simulink model "Q2"  (R2022b)
settings: Solver=VariableStepAuto  StartTime=0.0  StopTime=10.0  RelTol=1e-3
settings Model: Creator=Ali  LastModifiedBy=Ali

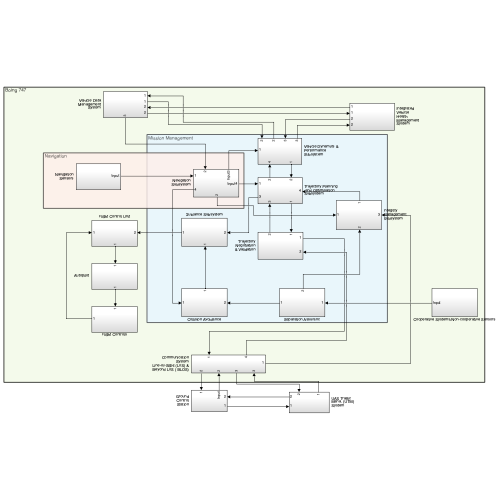
[thumbnail: Simulink's stored preview of the top-level diagram]
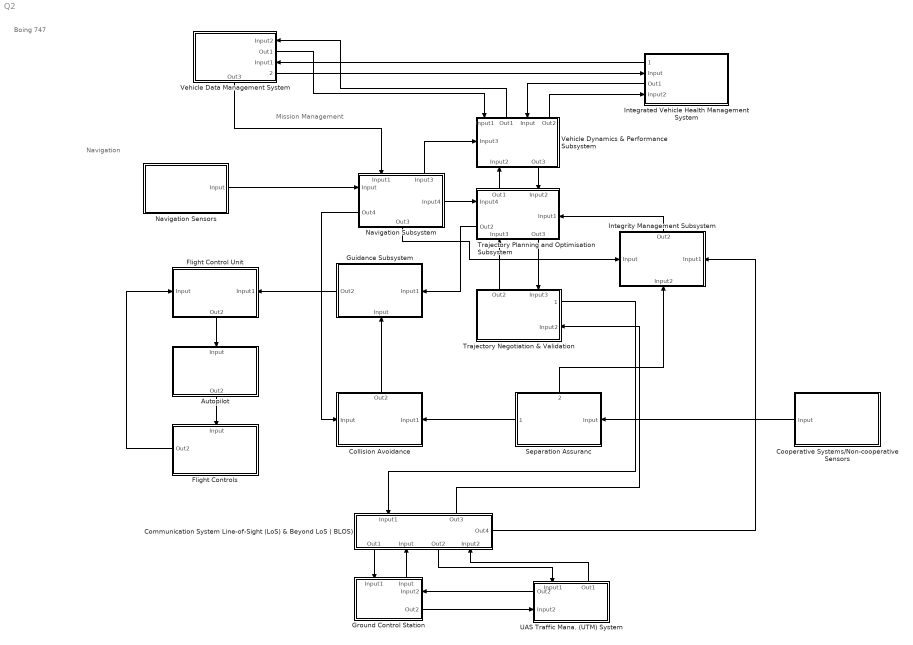
== system Q2 ==
  note: Mission Management
  note: Navigation
  note: Boing 747
  Autopilot : Subsystem
      settings: PortSchema="{\"entries\":[{\"content\":{\"sides\":[{\"content\":{\"connectorIds\":[]},\"type\":\"ConnectorPlacement.EquallySpacedRectSide\",\"uuid\":\"7c03228e-e6de-4210-83e4-dc60ea5d03ec\"},{\"content\":{\"connectorIds\":[],\"side\":\"RIGHT\"},\"type\":\"ConnectorPlacement.EquallySpacedRectSide\",\"uuid\":\"398f5b5b-7985-47d4-80b4-f710280625a6\"},{\"content\":{\"connectorIds\":[\"In1\"],\"side\":\"TOP\"},\"type\":\"ConnectorPlacement.EquallySpacedRectSide\",\"uuid\":\"212a440f-1f73-46c7-990f-e1425be29cd1\"},{\"content\":{\"connectorIds\":[\"Out1\"],\"side\":\"BOTTOM\"},\"type\":\"ConnectorPlacement.EquallySpacedRectSide\",\"uuid\":\"b57b75e4-92e7-45b5-b420-ccd9edaba603\"}]},\"type\":\"ConnectorPlacement.EquallySpacedConnector\",\"uuid\":\"cb83deef-b6b8-410a-b432-b2f3f2a9e8ae\"}],\"packageUris\":[\"http://schema.mathworks.com/mf0/Connector/R2020b\"],\"version\":\"1.0\"}"
  Collision Avoidance : Subsystem
      settings: PortSchema="{\"entries\":[{\"content\":{\"sides\":[{\"content\":{\"connectorIds\":[\"In1\"]},\"type\":\"ConnectorPlacement.EquallySpacedRectSide\",\"uuid\":\"8816de1e-4171-47af-bbd0-c7093bdd2ec4\"},{\"content\":{\"connectorIds\":[\"In2\"],\"side\":\"RIGHT\"},\"type\":\"ConnectorPlacement.EquallySpacedRectSide\",\"uuid\":\"4ec5b307-27a2-4754-b3e3-e34b35b208c2\"},{\"content\":{\"connectorIds\":[\"Out1\"],\"side\":\"TOP\"},\"type\":\"ConnectorPlacement.EquallySpacedRectSide\",\"uuid\":\"1be75602-f59e-4616-8d3b-3f7c07037b2b\"},{\"content\":{\"connectorIds\":[],\"side\":\"BOTTOM\"},\"type\":\"ConnectorPlacement.EquallySpacedRectSide\",\"uuid\":\"aaca4339-a36b-4f6c-91d5-5c0f7e0a86f3\"}]},\"type\":\"ConnectorPlacement.EquallySpacedConnector\",\"uuid\":\"f2ce33cf-07fa-49b4-80b6-e618028f6f8d\"}],\"packageUris\":[\"http://schema.mathworks.com/mf0/Connector/R2020b\"],\"version\":\"1.0\"}"
  Communication System Line-of-Sight (LoS) & Beyond LoS ( BLOS) : Subsystem
      settings: PortSchema="{\"entries\":[{\"content\":{\"sides\":[{\"content\":{\"connectorIds\":[]},\"type\":\"ConnectorPlacement.EquallySpacedRectSide\",\"uuid\":\"8816de1e-4171-47af-bbd0-c7093bdd2ec4\"},{\"content\":{\"connectorIds\":[\"Out1\"],\"side\":\"RIGHT\"},\"type\":\"ConnectorPlacement.EquallySpacedRectSide\",\"uuid\":\"4ec5b307-27a2-4754-b3e3-e34b35b208c2\"},{\"content\":{\"connectorIds\":[\"In1\",\"Out4\"],\"side\":\"TOP\"},\"type\":\"ConnectorPlacement.EquallySpacedRectSide\",\"uuid\":\"1be75602-f59e-4616-8d3b-3f7c07037b2b\"},{\"content\":{\"connectorIds\":[\"Out2\",\"In2\",\"Out3\",\"In3\"],\"side\":\"BOTTOM\"},\"type\":\"ConnectorPlacement.EquallySpacedRectSide\",\"uuid\":\"aaca4339-a36b-4f6c-91d5-5c0f7e0a86f3\"}]},\"type\":\"ConnectorPlacement.EquallySpacedConnector\",\"uuid\":\"f2ce33cf-07fa-49b4-80b6-e618028f6f8d\"}],\"packageUris\":[\"http://schema.mathworks.com/mf0/Connector/R2020b\"],\"version\":\"1.0\"}"
  Cooperative Systems/Non-cooperative Sensors : Subsystem
      settings: PortSchema="{\"entries\":[{\"content\":{\"sides\":[{\"content\":{\"connectorIds\":[\"Out1\"]},\"type\":\"ConnectorPlacement.EquallySpacedRectSide\",\"uuid\":\"8816de1e-4171-47af-bbd0-c7093bdd2ec4\"},{\"content\":{\"connectorIds\":[],\"side\":\"RIGHT\"},\"type\":\"ConnectorPlacement.EquallySpacedRectSide\",\"uuid\":\"4ec5b307-27a2-4754-b3e3-e34b35b208c2\"},{\"content\":{\"connectorIds\":[],\"side\":\"TOP\"},\"type\":\"ConnectorPlacement.EquallySpacedRectSide\",\"uuid\":\"1be75602-f59e-4616-8d3b-3f7c07037b2b\"},{\"content\":{\"connectorIds\":[],\"side\":\"BOTTOM\"},\"type\":\"ConnectorPlacement.EquallySpacedRectSide\",\"uuid\":\"aaca4339-a36b-4f6c-91d5-5c0f7e0a86f3\"}]},\"type\":\"ConnectorPlacement.EquallySpacedConnector\",\"uuid\":\"f2ce33cf-07fa-49b4-80b6-e618028f6f8d\"}],\"packageUris\":[\"http://schema.mathworks.com/mf0/Connector/R2020b\"],\"version\":\"1.0\"}"
  Flight Control Unit : Subsystem
      settings: PortSchema="{\"entries\":[{\"content\":{\"sides\":[{\"content\":{\"connectorIds\":[\"In1\"]},\"type\":\"ConnectorPlacement.EquallySpacedRectSide\",\"uuid\":\"7c03228e-e6de-4210-83e4-dc60ea5d03ec\"},{\"content\":{\"connectorIds\":[\"In2\"],\"side\":\"RIGHT\"},\"type\":\"ConnectorPlacement.EquallySpacedRectSide\",\"uuid\":\"398f5b5b-7985-47d4-80b4-f710280625a6\"},{\"content\":{\"connectorIds\":[],\"side\":\"TOP\"},\"type\":\"ConnectorPlacement.EquallySpacedRectSide\",\"uuid\":\"212a440f-1f73-46c7-990f-e1425be29cd1\"},{\"content\":{\"connectorIds\":[\"Out1\"],\"side\":\"BOTTOM\"},\"type\":\"ConnectorPlacement.EquallySpacedRectSide\",\"uuid\":\"b57b75e4-92e7-45b5-b420-ccd9edaba603\"}]},\"type\":\"ConnectorPlacement.EquallySpacedConnector\",\"uuid\":\"cb83deef-b6b8-410a-b432-b2f3f2a9e8ae\"}],\"packageUris\":[\"http://schema.mathworks.com/mf0/Connector/R2020b\"],\"version\":\"1.0\"}"
  Flight Controls : Subsystem
      settings: PortSchema="{\"entries\":[{\"content\":{\"sides\":[{\"content\":{\"connectorIds\":[\"Out1\"]},\"type\":\"ConnectorPlacement.EquallySpacedRectSide\",\"uuid\":\"7c03228e-e6de-4210-83e4-dc60ea5d03ec\"},{\"content\":{\"connectorIds\":[],\"side\":\"RIGHT\"},\"type\":\"ConnectorPlacement.EquallySpacedRectSide\",\"uuid\":\"398f5b5b-7985-47d4-80b4-f710280625a6\"},{\"content\":{\"connectorIds\":[\"In1\"],\"side\":\"TOP\"},\"type\":\"ConnectorPlacement.EquallySpacedRectSide\",\"uuid\":\"212a440f-1f73-46c7-990f-e1425be29cd1\"},{\"content\":{\"connectorIds\":[],\"side\":\"BOTTOM\"},\"type\":\"ConnectorPlacement.EquallySpacedRectSide\",\"uuid\":\"b57b75e4-92e7-45b5-b420-ccd9edaba603\"}]},\"type\":\"ConnectorPlacement.EquallySpacedConnector\",\"uuid\":\"cb83deef-b6b8-410a-b432-b2f3f2a9e8ae\"}],\"packageUris\":[\"http://schema.mathworks.com/mf0/Connector/R2020b\"],\"version\":\"1.0\"}"
  Ground Control Station : Subsystem
      settings: PortSchema="{\"entries\":[{\"content\":{\"sides\":[{\"content\":{\"connectorIds\":[]},\"type\":\"ConnectorPlacement.EquallySpacedRectSide\",\"uuid\":\"8816de1e-4171-47af-bbd0-c7093bdd2ec4\"},{\"content\":{\"connectorIds\":[\"In2\",\"Out1\"],\"side\":\"RIGHT\"},\"type\":\"ConnectorPlacement.EquallySpacedRectSide\",\"uuid\":\"4ec5b307-27a2-4754-b3e3-e34b35b208c2\"},{\"content\":{\"connectorIds\":[\"In1\",\"Out2\"],\"side\":\"TOP\"},\"type\":\"ConnectorPlacement.EquallySpacedRectSide\",\"uuid\":\"1be75602-f59e-4616-8d3b-3f7c07037b2b\"},{\"content\":{\"connectorIds\":[],\"side\":\"BOTTOM\"},\"type\":\"ConnectorPlacement.EquallySpacedRectSide\",\"uuid\":\"aaca4339-a36b-4f6c-91d5-5c0f7e0a86f3\"}]},\"type\":\"ConnectorPlacement.EquallySpacedConnector\",\"uuid\":\"f2ce33cf-07fa-49b4-80b6-e618028f6f8d\"}],\"packageUris\":[\"http://schema.mathworks.com/mf0/Connector/R2020b\"],\"version\":\"1.0\"}"
  Guidance Subsystem : Subsystem
      settings: PortSchema="{\"entries\":[{\"content\":{\"sides\":[{\"content\":{\"connectorIds\":[\"Out1\"]},\"type\":\"ConnectorPlacement.EquallySpacedRectSide\",\"uuid\":\"8816de1e-4171-47af-bbd0-c7093bdd2ec4\"},{\"content\":{\"connectorIds\":[\"In2\"],\"side\":\"RIGHT\"},\"type\":\"ConnectorPlacement.EquallySpacedRectSide\",\"uuid\":\"4ec5b307-27a2-4754-b3e3-e34b35b208c2\"},{\"content\":{\"connectorIds\":[],\"side\":\"TOP\"},\"type\":\"ConnectorPlacement.EquallySpacedRectSide\",\"uuid\":\"1be75602-f59e-4616-8d3b-3f7c07037b2b\"},{\"content\":{\"connectorIds\":[\"In1\"],\"side\":\"BOTTOM\"},\"type\":\"ConnectorPlacement.EquallySpacedRectSide\",\"uuid\":\"aaca4339-a36b-4f6c-91d5-5c0f7e0a86f3\"}]},\"type\":\"ConnectorPlacement.EquallySpacedConnector\",\"uuid\":\"f2ce33cf-07fa-49b4-80b6-e618028f6f8d\"}],\"packageUris\":[\"http://schema.mathworks.com/mf0/Connector/R2020b\"],\"version\":\"1.0\"}"
  Integrated Vehicle Health Management System : Subsystem
      settings: PortSchema="{\"entries\":[{\"content\":{\"sides\":[{\"content\":{\"connectorIds\":[\"Out1\",\"In1\",\"Out2\",\"In2\"]},\"type\":\"ConnectorPlacement.EquallySpacedRectSide\",\"uuid\":\"bd36125d-75c5-4143-b99c-3e4a87d10701\"},{\"content\":{\"connectorIds\":[],\"side\":\"RIGHT\"},\"type\":\"ConnectorPlacement.EquallySpacedRectSide\",\"uuid\":\"e6754b16-36a5-4be2-b98d-b46917597dce\"},{\"content\":{\"connectorIds\":[],\"side\":\"TOP\"},\"type\":\"ConnectorPlacement.EquallySpacedRectSide\",\"uuid\":\"193bbe33-aa7f-43da-961a-60435cc2b4dc\"},{\"content\":{\"connectorIds\":[],\"side\":\"BOTTOM\"},\"type\":\"ConnectorPlacement.EquallySpacedRectSide\",\"uuid\":\"1a0f7017-b5e6-4739-a088-f50189ea50e9\"}]},\"type\":\"ConnectorPlacement.EquallySpacedConnector\",\"uuid\":\"e77c47bd-b0a0-4c61-ab2d-e4f8b97a4182\"}],\"packageUris\":[\"http://schema.mathworks.com/mf0/Connector/R2020b\"],\"version\":\"1.0\"}"
  Integrity Management Subsystem : Subsystem
      settings: PortSchema="{\"entries\":[{\"content\":{\"sides\":[{\"content\":{\"connectorIds\":[\"In1\"]},\"type\":\"ConnectorPlacement.EquallySpacedRectSide\",\"uuid\":\"8816de1e-4171-47af-bbd0-c7093bdd2ec4\"},{\"content\":{\"connectorIds\":[\"In3\"],\"side\":\"RIGHT\"},\"type\":\"ConnectorPlacement.EquallySpacedRectSide\",\"uuid\":\"4ec5b307-27a2-4754-b3e3-e34b35b208c2\"},{\"content\":{\"connectorIds\":[\"Out1\"],\"side\":\"TOP\"},\"type\":\"ConnectorPlacement.EquallySpacedRectSide\",\"uuid\":\"1be75602-f59e-4616-8d3b-3f7c07037b2b\"},{\"content\":{\"connectorIds\":[\"In2\"],\"side\":\"BOTTOM\"},\"type\":\"ConnectorPlacement.EquallySpacedRectSide\",\"uuid\":\"aaca4339-a36b-4f6c-91d5-5c0f7e0a86f3\"}]},\"type\":\"ConnectorPlacement.EquallySpacedConnector\",\"uuid\":\"f2ce33cf-07fa-49b4-80b6-e618028f6f8d\"}],\"packageUris\":[\"http://schema.mathworks.com/mf0/Connector/R2020b\"],\"version\":\"1.0\"}"
  Navigation Subsystem : Subsystem
      settings: PortSchema="{\"entries\":[{\"content\":{\"sides\":[{\"content\":{\"connectorIds\":[\"In1\",\"Out4\"]},\"type\":\"ConnectorPlacement.EquallySpacedRectSide\",\"uuid\":\"8816de1e-4171-47af-bbd0-c7093bdd2ec4\"},{\"content\":{\"connectorIds\":[\"Out1\"],\"side\":\"RIGHT\"},\"type\":\"ConnectorPlacement.EquallySpacedRectSide\",\"uuid\":\"4ec5b307-27a2-4754-b3e3-e34b35b208c2\"},{\"content\":{\"connectorIds\":[\"In2\",\"Out3\"],\"side\":\"TOP\"},\"type\":\"ConnectorPlacement.EquallySpacedRectSide\",\"uuid\":\"1be75602-f59e-4616-8d3b-3f7c07037b2b\"},{\"content\":{\"connectorIds\":[\"Out2\"],\"side\":\"BOTTOM\"},\"type\":\"ConnectorPlacement.EquallySpacedRectSide\",\"uuid\":\"aaca4339-a36b-4f6c-91d5-5c0f7e0a86f3\"}]},\"type\":\"ConnectorPlacement.EquallySpacedConnector\",\"uuid\":\"f2ce33cf-07fa-49b4-80b6-e618028f6f8d\"}],\"packageUris\":[\"http://schema.mathworks.com/mf0/Connector/R2020b\"],\"version\":\"1.0\"}"
  Navigation Sensors : Subsystem
  Separation Assuranc : Subsystem
      settings: PortSchema="{\"entries\":[{\"content\":{\"sides\":[{\"content\":{\"connectorIds\":[\"Out2\"]},\"type\":\"ConnectorPlacement.EquallySpacedRectSide\",\"uuid\":\"8816de1e-4171-47af-bbd0-c7093bdd2ec4\"},{\"content\":{\"connectorIds\":[\"In1\"],\"side\":\"RIGHT\"},\"type\":\"ConnectorPlacement.EquallySpacedRectSide\",\"uuid\":\"4ec5b307-27a2-4754-b3e3-e34b35b208c2\"},{\"content\":{\"connectorIds\":[\"Out1\"],\"side\":\"TOP\"},\"type\":\"ConnectorPlacement.EquallySpacedRectSide\",\"uuid\":\"1be75602-f59e-4616-8d3b-3f7c07037b2b\"},{\"content\":{\"connectorIds\":[],\"side\":\"BOTTOM\"},\"type\":\"ConnectorPlacement.EquallySpacedRectSide\",\"uuid\":\"aaca4339-a36b-4f6c-91d5-5c0f7e0a86f3\"}]},\"type\":\"ConnectorPlacement.EquallySpacedConnector\",\"uuid\":\"f2ce33cf-07fa-49b4-80b6-e618028f6f8d\"}],\"packageUris\":[\"http://schema.mathworks.com/mf0/Connector/R2020b\"],\"version\":\"1.0\"}"
  Trajectory Negotiation & Validation : Subsystem
      settings: PortSchema="{\"entries\":[{\"content\":{\"sides\":[{\"content\":{\"connectorIds\":[]},\"type\":\"ConnectorPlacement.EquallySpacedRectSide\",\"uuid\":\"bd36125d-75c5-4143-b99c-3e4a87d10701\"},{\"content\":{\"connectorIds\":[\"Out1\",\"In2\"],\"side\":\"RIGHT\"},\"type\":\"ConnectorPlacement.EquallySpacedRectSide\",\"uuid\":\"e6754b16-36a5-4be2-b98d-b46917597dce\"},{\"content\":{\"connectorIds\":[\"Out2\",\"In1\"],\"side\":\"TOP\"},\"type\":\"ConnectorPlacement.EquallySpacedRectSide\",\"uuid\":\"193bbe33-aa7f-43da-961a-60435cc2b4dc\"},{\"content\":{\"connectorIds\":[],\"side\":\"BOTTOM\"},\"type\":\"ConnectorPlacement.EquallySpacedRectSide\",\"uuid\":\"1a0f7017-b5e6-4739-a088-f50189ea50e9\"}]},\"type\":\"ConnectorPlacement.EquallySpacedConnector\",\"uuid\":\"e77c47bd-b0a0-4c61-ab2d-e4f8b97a4182\"}],\"packageUris\":[\"http://schema.mathworks.com/mf0/Connector/R2020b\"],\"version\":\"1.0\"}"
  Trajectory Planning and Optimisation Subsystem : Subsystem
      settings: PortSchema="{\"entries\":[{\"content\":{\"sides\":[{\"content\":{\"connectorIds\":[\"In1\",\"Out3\"]},\"type\":\"ConnectorPlacement.EquallySpacedRectSide\",\"uuid\":\"bd36125d-75c5-4143-b99c-3e4a87d10701\"},{\"content\":{\"connectorIds\":[\"In4\"],\"side\":\"RIGHT\"},\"type\":\"ConnectorPlacement.EquallySpacedRectSide\",\"uuid\":\"e6754b16-36a5-4be2-b98d-b46917597dce\"},{\"content\":{\"connectorIds\":[\"Out2\",\"In2\"],\"side\":\"TOP\"},\"type\":\"ConnectorPlacement.EquallySpacedRectSide\",\"uuid\":\"193bbe33-aa7f-43da-961a-60435cc2b4dc\"},{\"content\":{\"connectorIds\":[\"In3\",\"Out1\"],\"side\":\"BOTTOM\"},\"type\":\"ConnectorPlacement.EquallySpacedRectSide\",\"uuid\":\"1a0f7017-b5e6-4739-a088-f50189ea50e9\"}]},\"type\":\"ConnectorPlacement.EquallySpacedConnector\",\"uuid\":\"e77c47bd-b0a0-4c61-ab2d-e4f8b97a4182\"}],\"packageUris\":[\"http://schema.mathworks.com/mf0/Connector/R2020b\"],\"version\":\"1.0\"}"
  UAS Traffic Mana. (UTM) System : Subsystem
      settings: PortSchema="{\"entries\":[{\"content\":{\"sides\":[{\"content\":{\"connectorIds\":[\"Out2\",\"In1\"]},\"type\":\"ConnectorPlacement.EquallySpacedRectSide\",\"uuid\":\"8816de1e-4171-47af-bbd0-c7093bdd2ec4\"},{\"content\":{\"connectorIds\":[],\"side\":\"RIGHT\"},\"type\":\"ConnectorPlacement.EquallySpacedRectSide\",\"uuid\":\"4ec5b307-27a2-4754-b3e3-e34b35b208c2\"},{\"content\":{\"connectorIds\":[\"In2\",\"Out1\"],\"side\":\"TOP\"},\"type\":\"ConnectorPlacement.EquallySpacedRectSide\",\"uuid\":\"1be75602-f59e-4616-8d3b-3f7c07037b2b\"},{\"content\":{\"connectorIds\":[],\"side\":\"BOTTOM\"},\"type\":\"ConnectorPlacement.EquallySpacedRectSide\",\"uuid\":\"aaca4339-a36b-4f6c-91d5-5c0f7e0a86f3\"}]},\"type\":\"ConnectorPlacement.EquallySpacedConnector\",\"uuid\":\"f2ce33cf-07fa-49b4-80b6-e618028f6f8d\"}],\"packageUris\":[\"http://schema.mathworks.com/mf0/Connector/R2020b\"],\"version\":\"1.0\"}"
  Vehicle Data Management System : Subsystem
      settings: PortSchema="{\"entries\":[{\"content\":{\"sides\":[{\"content\":{\"connectorIds\":[]},\"type\":\"ConnectorPlacement.EquallySpacedRectSide\",\"uuid\":\"bd36125d-75c5-4143-b99c-3e4a87d10701\"},{\"content\":{\"connectorIds\":[\"In1\",\"Out1\",\"In2\",\"Out2\"],\"side\":\"RIGHT\"},\"type\":\"ConnectorPlacement.EquallySpacedRectSide\",\"uuid\":\"e6754b16-36a5-4be2-b98d-b46917597dce\"},{\"content\":{\"connectorIds\":[],\"side\":\"TOP\"},\"type\":\"ConnectorPlacement.EquallySpacedRectSide\",\"uuid\":\"193bbe33-aa7f-43da-961a-60435cc2b4dc\"},{\"content\":{\"connectorIds\":[\"Out3\"],\"side\":\"BOTTOM\"},\"type\":\"ConnectorPlacement.EquallySpacedRectSide\",\"uuid\":\"1a0f7017-b5e6-4739-a088-f50189ea50e9\"}]},\"type\":\"ConnectorPlacement.EquallySpacedConnector\",\"uuid\":\"e77c47bd-b0a0-4c61-ab2d-e4f8b97a4182\"}],\"packageUris\":[\"http://schema.mathworks.com/mf0/Connector/R2020b\"],\"version\":\"1.0\"}"
  Vehicle Dynamics & Performance Subsystem : Subsystem
      settings: PortSchema="{\"entries\":[{\"content\":{\"sides\":[{\"content\":{\"connectorIds\":[\"In1\"]},\"type\":\"ConnectorPlacement.EquallySpacedRectSide\",\"uuid\":\"bd36125d-75c5-4143-b99c-3e4a87d10701\"},{\"content\":{\"connectorIds\":[],\"side\":\"RIGHT\"},\"type\":\"ConnectorPlacement.EquallySpacedRectSide\",\"uuid\":\"e6754b16-36a5-4be2-b98d-b46917597dce\"},{\"content\":{\"connectorIds\":[\"In2\",\"Out2\",\"In3\",\"Out3\"],\"side\":\"TOP\"},\"type\":\"ConnectorPlacement.EquallySpacedRectSide\",\"uuid\":\"193bbe33-aa7f-43da-961a-60435cc2b4dc\"},{\"content\":{\"connectorIds\":[\"In4\",\"Out1\"],\"side\":\"BOTTOM\"},\"type\":\"ConnectorPlacement.EquallySpacedRectSide\",\"uuid\":\"1a0f7017-b5e6-4739-a088-f50189ea50e9\"}]},\"type\":\"ConnectorPlacement.EquallySpacedConnector\",\"uuid\":\"e77c47bd-b0a0-4c61-ab2d-e4f8b97a4182\"}],\"packageUris\":[\"http://schema.mathworks.com/mf0/Connector/R2020b\"],\"version\":\"1.0\"}"
  wires:
  Vehicle Dynamics & Performance Subsystem/3(Out2) -> Integrated Vehicle Health Management System/2(Input2)
  Integrated Vehicle Health Management System/2(Out1) -> Vehicle Dynamics & Performance Subsystem/3(Input)
  Vehicle Dynamics & Performance Subsystem/2(Out1) -> Vehicle Data Management System/1(Input2)
  Vehicle Data Management System/1(Out1) -> Vehicle Dynamics & Performance Subsystem/2(Input1)
  Vehicle Dynamics & Performance Subsystem/1(Out3) -> Trajectory Planning and Optimisation Subsystem/2(Input2)
  Trajectory Planning and Optimisation Subsystem/2(Out1) -> Vehicle Dynamics & Performance Subsystem/4(Input2)
  Navigation Subsystem/1(Input4) -> Trajectory Planning and Optimisation Subsystem/1(Input4)
  Navigation Subsystem/3(Input3) -> Vehicle Dynamics & Performance Subsystem/1(Input3)
  Vehicle Data Management System/3(Out3) -> Navigation Subsystem/2(Input1)
  Trajectory Planning and Optimisation Subsystem/3(Out2) -> Guidance Subsystem/2(Input1)
  Navigation Subsystem/2(Out3) -> Integrity Management Subsystem/1(Input)
  Navigation Sensors/1(Input) -> Navigation Subsystem/1(Input)
  Navigation Subsystem/4(Out4) -> Collision Avoidance/1(Input)
  Guidance Subsystem/1(Out2) -> Flight Control Unit/2(Input1)
  Flight Controls/1(Out2) -> Flight Control Unit/1(Input)
  Flight Control Unit/1(Out2) -> Autopilot/1(Input)
  Autopilot/1(Out2) -> Flight Controls/1(Input)
  Collision Avoidance/1(Out2) -> Guidance Subsystem/1(Input)
  Separation Assuranc/2(1) -> Collision Avoidance/2(Input1)
  Separation Assuranc/1(2) -> Integrity Management Subsystem/2(Input2)
  Cooperative Systems/Non-cooperative Sensors/1(Input) -> Separation Assuranc/1(Input)
  Ground Control Station/2(Input) -> Communication System Line-of-Sight (LoS) & Beyond LoS ( BLOS)/2(Input)
  Communication System Line-of-Sight (LoS) & Beyond LoS ( BLOS)/2(Out1) -> Ground Control Station/1(Input1)
  Communication System Line-of-Sight (LoS) & Beyond LoS ( BLOS)/3(Out2) -> UAS Traffic Mana. (UTM) System/2(Input1)
  UAS Traffic Mana. (UTM) System/1(Out1) -> Communication System Line-of-Sight (LoS) & Beyond LoS ( BLOS)/3(Input2)
  UAS Traffic Mana. (UTM) System/2(Out2) -> Ground Control Station/2(Input2)
  Ground Control Station/1(Out2) -> UAS Traffic Mana. (UTM) System/1(Input2)
  Communication System Line-of-Sight (LoS) & Beyond LoS ( BLOS)/4(Out3) -> Trajectory Negotiation & Validation/2(Input2)
  Trajectory Negotiation & Validation/1(1) -> Communication System Line-of-Sight (LoS) & Beyond LoS ( BLOS)/1(Input1)
  Trajectory Planning and Optimisation Subsystem/1(Out3) -> Trajectory Negotiation & Validation/1(Input3)
  Trajectory Negotiation & Validation/2(Out2) -> Trajectory Planning and Optimisation Subsystem/3(Input3)
  Vehicle Data Management System/2(2) -> Integrated Vehicle Health Management System/1(Input)
  Communication System Line-of-Sight (LoS) & Beyond LoS ( BLOS)/1(Out4) -> Integrity Management Subsystem/3(Input1)
  Integrity Management Subsystem/1(Out2) -> Trajectory Planning and Optimisation Subsystem/4(Input1)
  Integrated Vehicle Health Management System/1(1) -> Vehicle Data Management System/2(Input1)

== system Q2/Autopilot ==
  Input : Inport
  Out2 : Outport
  wires:
  Input/1 -> Out2/1

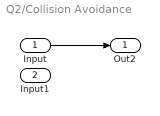
== system Q2/Collision Avoidance ==
  Input : Inport
  Input1 : Inport  Port=2
  Out2 : Outport
  wires:
  Input/1 -> Out2/1

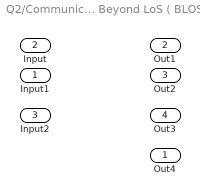
== system Q2/Communication System Line-of-Sight (LoS) & Beyond LoS ( BLOS) ==
  Input1 : Inport
  Input : Inport  Port=2
  Input2 : Inport  Port=3
  Out4 : Outport
  Out1 : Outport  Port=2
  Out2 : Outport  Port=3
  Out3 : Outport  Port=4

== system Q2/Cooperative Systems//Non-cooperative Sensors ==
  Input : Outport

== system Q2/Flight Control Unit ==
  Input : Inport
  Input1 : Inport  Port=2
  Out2 : Outport
  wires:
  Input/1 -> Out2/1

== system Q2/Flight Controls ==
  Input : Inport
  Out2 : Outport
  wires:
  Input/1 -> Out2/1

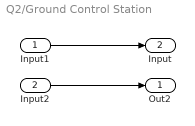
== system Q2/Ground Control Station ==
  Input1 : Inport
  Input2 : Inport  Port=2
  Out2 : Outport
  Input : Outport  Port=2
  wires:
  Input1/1 -> Input/1
  Input2/1 -> Out2/1

== system Q2/Guidance Subsystem ==
  Input : Inport
  Input1 : Inport  Port=2
  Out2 : Outport
  wires:
  Input/1 -> Out2/1

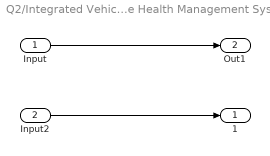
== system Q2/Integrated Vehicle Health Management System ==
  Input : Inport
  Input2 : Inport  Port=2
  1 : Outport
  Out1 : Outport  Port=2
  wires:
  Input/1 -> Out1/1
  Input2/1 -> 1/1

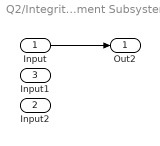
== system Q2/Integrity Management Subsystem ==
  Input : Inport
  Input2 : Inport  Port=2
  Input1 : Inport  Port=3
  Out2 : Outport
  wires:
  Input/1 -> Out2/1

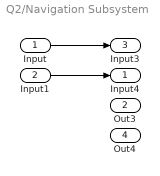
== system Q2/Navigation Subsystem ==
  Input : Inport
  Input1 : Inport  Port=2
  Input4 : Outport
  Out3 : Outport  Port=2
  Input3 : Outport  Port=3
  Out4 : Outport  Port=4
  wires:
  Input1/1 -> Input4/1
  Input/1 -> Input3/1

== system Q2/Navigation Sensors ==
  Input : Outport

== system Q2/Separation Assuranc ==
  Input : Inport
  2 : Outport
  1 : Outport  Port=2
  wires:
  Input/1 -> 1/1

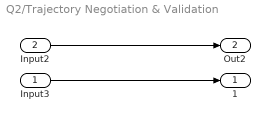
== system Q2/Trajectory Negotiation & Validation ==
  Input3 : Inport
  Input2 : Inport  Port=2
  1 : Outport
  Out2 : Outport  Port=2
  wires:
  Input2/1 -> Out2/1
  Input3/1 -> 1/1

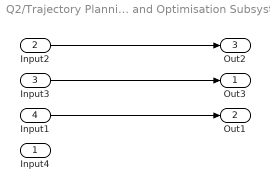
== system Q2/Trajectory Planning and Optimisation Subsystem ==
  Input4 : Inport
  Input2 : Inport  Port=2
  Input3 : Inport  Port=3
  Input1 : Inport  Port=4
  Out3 : Outport
  Out1 : Outport  Port=2
  Out2 : Outport  Port=3
  wires:
  Input2/1 -> Out2/1
  Input3/1 -> Out3/1
  Input1/1 -> Out1/1

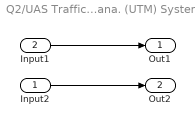
== system Q2/UAS Traffic Mana. (UTM) System ==
  Input2 : Inport
  Input1 : Inport  Port=2
  Out1 : Outport
  Out2 : Outport  Port=2
  wires:
  Input1/1 -> Out1/1
  Input2/1 -> Out2/1

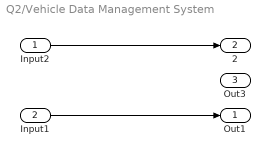
== system Q2/Vehicle Data Management System ==
  Input2 : Inport
  Input1 : Inport  Port=2
  Out1 : Outport
  2 : Outport  Port=2
  Out3 : Outport  Port=3
  wires:
  Input2/1 -> 2/1
  Input1/1 -> Out1/1

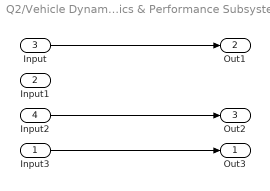
== system Q2/Vehicle Dynamics & Performance Subsystem ==
  Input3 : Inport
  Input1 : Inport  Port=2
  Input : Inport  Port=3
  Input2 : Inport  Port=4
  Out3 : Outport
  Out1 : Outport  Port=2
  Out2 : Outport  Port=3
  wires:
  Input/1 -> Out1/1
  Input2/1 -> Out2/1
  Input3/1 -> Out3/1
